simulink model "Simulink_Model_for_Problem_Set_1"  (Simulink 8.7)
settings: Solver=FixedStepAuto  StartTime=0.0  StopTime=280  FixedStep=0.07  RelTol=1e-3
settings Model: Creator=hjpeter  LastModifiedBy=eispin
settings DataIOCC: LimitDataPoints=off  SignalLoggingSaveFormat=ModelDataLogs  SaveOutput=off  SaveTime=off
settings OptimizationCC: ExpressionDepthLimit=2147483647
settings DebuggingCC: SolverPrmCheckMsg=warning  FcnCallInpInsideContextMsg=UseLocalSettings  StateNameClashWarn=warning
settings GRTTargetCC: CombineOutputUpdateFcns=off  GRTInterface=on
settings ConfigComp: CovSFcnEnable=off

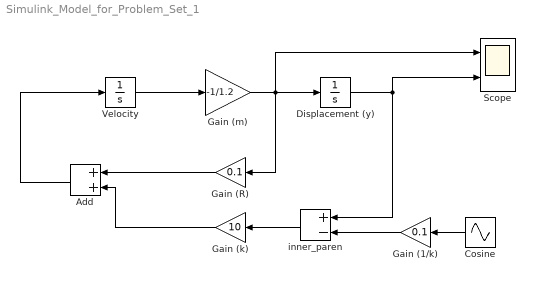
== system Simulink_Model_for_Problem_Set_1 ==
  Add : Sum
  Cosine : Sin  Frequency=0.5*(2*pi)  Phase=pi/2  SampleTime=0
  Displacement (y) : Integrator  InitialCondition=15
  Gain (1/k) : Gain  Gain=0.1
  Gain (R) : Gain  Gain=0.1
  Gain (k) : Gain  Gain=10
  Gain (m) : Gain  Gain=-1/1.2
  Scope : Scope  NumInputPorts=2
  Velocity : Integrator
  inner_paren : Sum  Inputs=+-
  wires:
  Displacement (y)/1 -> inner_paren/1, Scope/2
  Velocity/1 -> Gain (m)/1
  Gain (m)/1 -> Displacement (y)/1, Gain (R)/1, Scope/1
  Gain (R)/1 -> Add/1
  Gain (k)/1 -> Add/2
  Add/1 -> Velocity/1
  inner_paren/1 -> Gain (k)/1
  Gain (1/k)/1 -> inner_paren/2
  Cosine/1 -> Gain (1/k)/1
